simulink model "Control_MIMO_LTI_V2017"  (R2017a)
settings: Solver=VariableStepAuto  StartTime=0.0  StopTime=tsim  MaxStep=0.01  RelTol=1e-3
values from neighbouring files (symbols this model uses):
  L = tau/1000    [AlocaPID.m]
  s1 = 100    [Control_MIMO_WaB.m]
  s2 = 50    [Control_MIMO_WaB.m]
  ts1 = 5    [Control_MIMO_WaB.m]
  ts2 = 80    [Control_MIMO_WaB.m]
undefined symbols (not defined in the file or in its folder): R
libraries: cstblocks x4
settings Model: Creator=Sergio  LastModifiedBy=Sergio

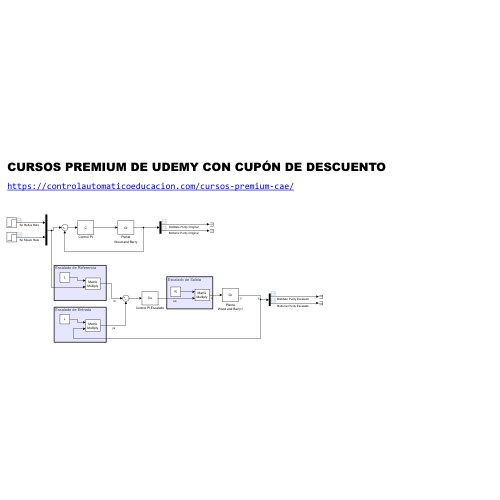
[thumbnail: Simulink's stored preview of the top-level diagram]
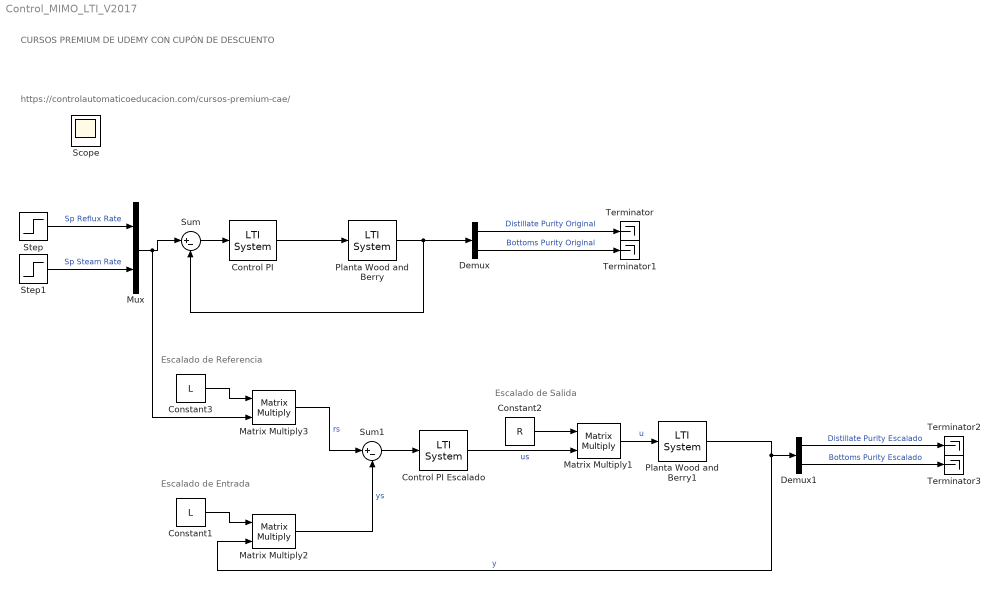
== system Control_MIMO_LTI_V2017 ==
  note: https://controlautomaticoeducacion.com/cursos-premium-cae/
  note: CURSOS PREMIUM DE UDEMY CON CUPÓN DE DESCUENTO
  note: Escalado de Entrada
  note: Escalado de Salida
  note: Escalado de Referencia
  Constant1 : Constant  Value=L
  Constant2 : Constant  Value=R
  Constant3 : Constant  Value=L
  Control PI : cstblocks/LTI System  sys=C  IC=[]
  Control PI Escalado : cstblocks/LTI System  sys=Ce  IC=[]
  Demux : Demux  Outputs=2
  Demux1 : Demux  Outputs=2
  Matrix Multiply1 : Product  Multiplication=Matrix(*)
  Matrix Multiply2 : Product  Multiplication=Matrix(*)
  Matrix Multiply3 : Product  Multiplication=Matrix(*)
  Mux : Mux  Inputs=2
  Planta Wood and Berry : cstblocks/LTI System  sys=Gr  IC=[]
  Planta Wood and Berry1 : cstblocks/LTI System  sys=Gr  IC=[]
  Step : Step  Time=ts1  After=s1  SampleTime=0
  Step1 : Step  Time=ts2  After=s2  SampleTime=0
  Sum : Sum  Inputs=|+-
  Sum1 : Sum  Inputs=|+-
  Terminator{,1..3} (4 alike) : Terminator
  Scope : Scope
  wires:
  Step/1 -> Mux/1  "Sp Reflux Rate"
  Step1/1 -> Mux/2  "Sp Steam Rate"
  Sum/1 -> Control PI/1
  Planta Wood and Berry/1 -> Demux/1, Sum/2
  Demux/1 -> Terminator/1  "Distillate Purity Original"
  Demux/2 -> Terminator1/1  "Bottoms Purity Original"
  Constant1/1 -> Matrix Multiply2/1
  Control PI Escalado/1 -> Matrix Multiply1/2  "us"
  Constant2/1 -> Matrix Multiply1/1
  Matrix Multiply1/1 -> Planta Wood and Berry1/1  "u"
  Demux1/2 -> Terminator3/1  "Bottoms Purity Escalado"
  Demux1/1 -> Terminator2/1  "Distillate Purity Escalado"
  Mux/1 -> Matrix Multiply3/2, Sum/1
  Constant3/1 -> Matrix Multiply3/1
  Matrix Multiply2/1 -> Sum1/2  "ys"
  Matrix Multiply3/1 -> Sum1/1  "rs"
  Sum1/1 -> Control PI Escalado/1
  Control PI/1 -> Planta Wood and Berry/1
  Planta Wood and Berry1/1 -> Matrix Multiply2/2, Demux1/1  "y"
